simulink model "model_main"  (R2020b)
settings: Solver=VariableStepAuto  StartTime=0.0  StopTime=100.0  RelTol=1e-3
libraries: sharedtransform x1
settings Model: Creator=Dogukan  LastModifiedBy=dogukan

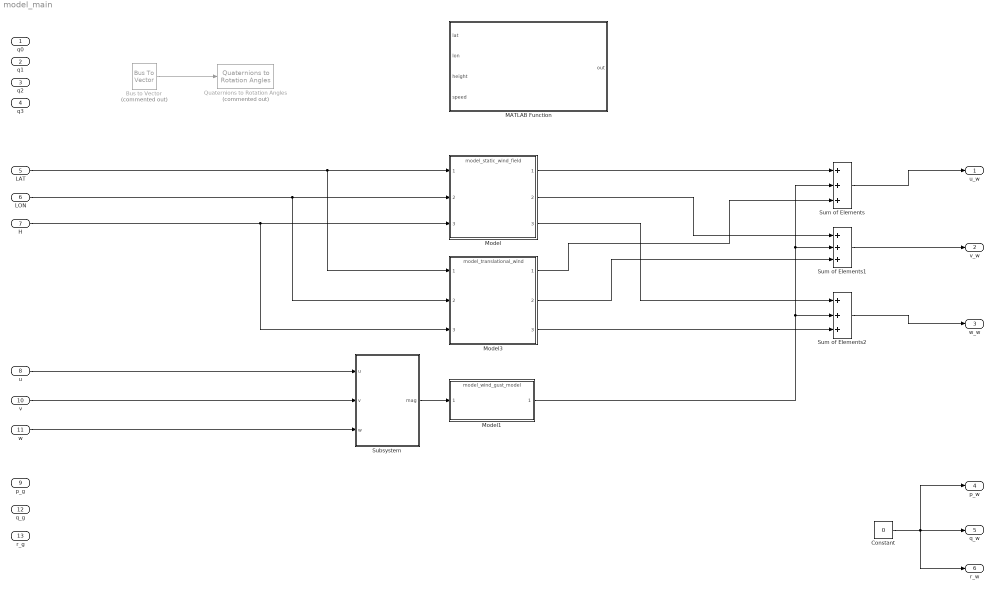
== system model_main ==
  q0 : Inport
  q1 : Inport  Port=2
  q2 : Inport  Port=3
  q3 : Inport  Port=4
  LAT : Inport  Port=5
  LON : Inport  Port=6
  H : Inport  Port=7
  u : Inport  Port=8  OutDataTypeStr=double
  p_g : Inport  Port=9  OutDataTypeStr=double
  v : Inport  Port=10  OutDataTypeStr=double
  w : Inport  Port=11  OutDataTypeStr=double
  q_g : Inport  Port=12  OutDataTypeStr=double
  r_g : Inport  Port=13  OutDataTypeStr=double
  Bus to Vector : BusToVector  Commented=on
  Constant : Constant  Value=0
  MATLAB Function : MATLAB Function  TreatAsAtomicUnit=on
  Model : ModelReference  ModelNameDialog=model_static_wind_field.slx  SimulationMode=Normal  ModelReferenceVersion=1.29
  Model1 : ModelReference  ModelNameDialog=model_wind_gust_model.slx  SimulationMode=Normal  ModelReferenceVersion=1.4
  Model3 : ModelReference  ModelNameDialog=model_translational_wind.slx  SimulationMode=Normal  ModelReferenceVersion=1.10
  Quaternions to Rotation Angles : sharedtransform/Quaternions to Rotation Angles  Commented=on  rotationOrder=ZYX  aMode=aMode
      settings: SourceProductBaseCode=AE,PW,MT,UV,VE,VP
  Subsystem : Subsystem
  Sum of Elements : Sum  Inputs=+++
  Sum of Elements1 : Sum  Inputs=+++
  Sum of Elements2 : Sum  Inputs=+++
  u_w : Outport  SignalName=u_w  OutDataTypeStr=double
  v_w : Outport  Port=2  SignalName=v_w  OutDataTypeStr=double
  w_w : Outport  Port=3  SignalName=w_w  OutDataTypeStr=double
  p_w : Outport  Port=4  SignalName=p_w  OutDataTypeStr=double
  q_w : Outport  Port=5  SignalName=q_w  OutDataTypeStr=double
  r_w : Outport  Port=6  SignalName=r_w  OutDataTypeStr=double
  wires:
  LAT/1 -> Model3/1, Model/1
  LON/1 -> Model3/2, Model/2
  H/1 -> Model3/3, Model/3
  Constant/1 -> q_w/1, p_w/1, r_w/1
  Bus to Vector/1 -> Quaternions to Rotation Angles/1
  Model/2 -> Sum of Elements1/1
  Model/3 -> Sum of Elements2/1
  Subsystem/1(mag) -> Model1/1
  Model/1 -> Sum of Elements/1
  Model1/1 -> Sum of Elements/2, Sum of Elements1/2, Sum of Elements2/2
  Sum of Elements/1 -> u_w/1
  Sum of Elements1/1 -> v_w/1
  Sum of Elements2/1 -> w_w/1
  Model3/1 -> Sum of Elements/3
  Model3/2 -> Sum of Elements1/3
  Model3/3 -> Sum of Elements2/3
  u/1 -> Subsystem/1(u)
  v/1 -> Subsystem/2(v)
  w/1 -> Subsystem/3(w)

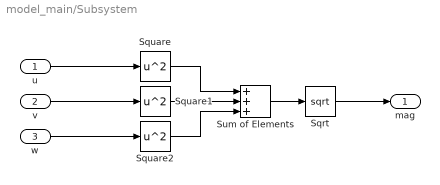
== system model_main/Subsystem ==
  u : Inport  OutDataTypeStr=double
  v : Inport  Port=2  OutDataTypeStr=double
  w : Inport  Port=3  OutDataTypeStr=double
  Sqrt : Sqrt  SaturateOnIntegerOverflow=on
  Square : Math  Operator=square  SaturateOnIntegerOverflow=on
  Square1 : Math  Operator=square  SaturateOnIntegerOverflow=on
  Square2 : Math  Operator=square  SaturateOnIntegerOverflow=on
  Sum of Elements : Sum  Inputs=+++
  mag : Outport
  wires:
  Sqrt/1 -> mag/1
  u/1 -> Square/1
  w/1 -> Square2/1
  v/1 -> Square1/1
  Square/1 -> Sum of Elements/1
  Square1/1 -> Sum of Elements/2
  Square2/1 -> Sum of Elements/3
  Sum of Elements/1 -> Sqrt/1

== matlab function model_main/MATLAB Function ==
  data: lat input; out output; lon input; height input; speed input
function out = generateWindNearby(lat, lon, height, speed)
    rng(datetime);

    % TODO: Look into MIL-F Spec
    % TODO: Maybe inline this so association becomes clearer
    amplitude = x*rand;
    width = y*rand;

    sinusoidal_gust{length(sinusoidal_gust)+1} = createSinusoidalGust(...
        5, ...
        createBoundaries(), ...
        amplitude, ...
        width, ...
        speed);

    trapezoidal_gust{length(trapezoidal_gust)+1} = createTrapezoidalGust(...
        createBoundaries(), ...
        pi/4, ...
        pi/4, ...
        amplitude, ...
        width);
end
